simulink model "handone_simulink_2018b"  (R2018b)
settings: Solver=ode1  StartTime=0.0  StopTime=5  FixedStep=1e-3  RelTol=1e-3
model workspace: external: MAT-File D:\repos\hand_modeling_toolbox\examples\hand_one\hand_one_model.mat (data not in the file)
values from neighbouring files (symbols this model uses):
  d_coupling = 1e-5    (= 1e-05)    [hand_one_PTI.m]
  D_j = 1e-4 * [1,1,1,1]'    [hand_one_PTI.m]    (also in hand_one_model.m = 0* 1e-5 * [1,1,1,1]')
  finger_handone = init_from_rst(finger_urdf)    [hand_one_PTI.m]    (also in hand_one_model.m)
  k_coupling = 1e-1    (= 0.1)    [hand_one_PTI.m]
  mdh_matrix = mdh_struct_to_matrix(mdh_ori,1)    [create_handone_finger_from_urdf.m]    (also in hand_one_PTI.m; hand_one_model.m)
  q_init = [0.2,0.2]'    [create_hand_one_finger.m]    (also in hand_one_PTI.m = [0,0,0,0]'; hand_one_model.m = [0,0,0.1,0]')
  q_stiff_init = [0,0,0,0]'    [hand_one_PTI.m]    (also in hand_one_model.m)
  qD_init = [0,0,0,0]'    [hand_one_PTI.m]    (also in hand_one_model.m)
  S_j = 1e-4 * [1,1,1,1]'    [hand_one_PTI.m]    (also in hand_one_model.m = 0* 1e-4 * [1,1,1,1]')
undefined symbols (not defined in the file or in its folder): q_desired
libraries: unity_lib_UDP x1
settings Model: Creator=ge26jow  LastModifiedBy=ge26jow
settings DataIOCC: ReturnWorkspaceOutputs=on
settings DebuggingCC: SFMachineParentedDataDiag=error

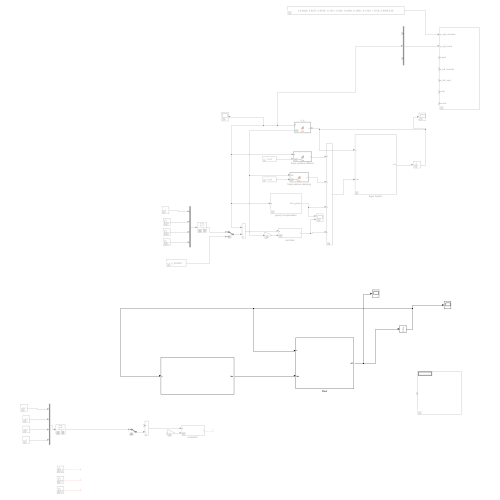
[thumbnail: Simulink's stored preview of the top-level diagram]
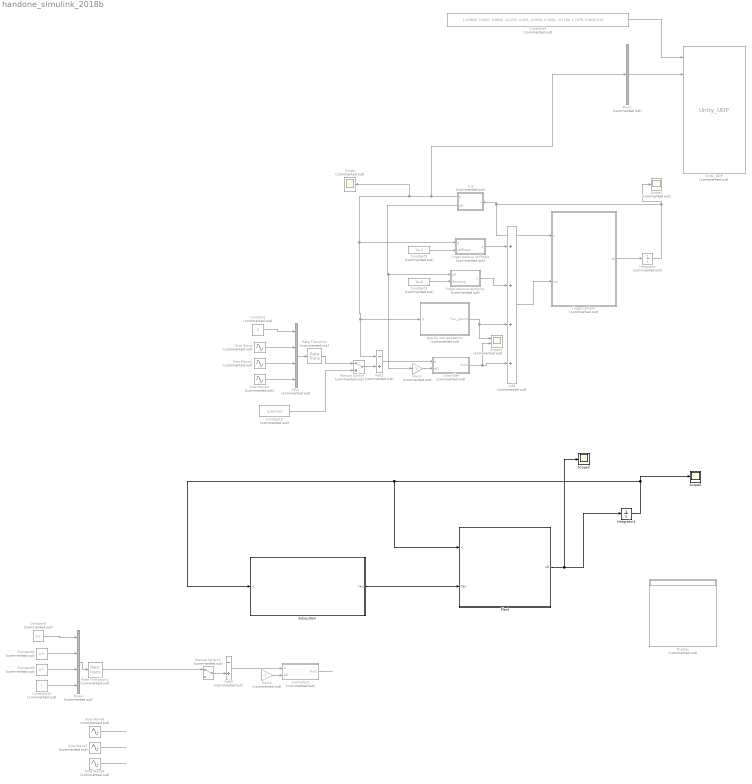
== system handone_simulink_2018b ==
  Add : Sum  Commented=on  Inputs=++++
  Add1 : Sum  Commented=on  Inputs=-+
  Add3 : Sum  Commented=on  Inputs=-+
  Constant : Constant  Commented=on  Value=0
  Constant1 : Constant  Commented=on  Value=1e-4
  Constant10 : Constant  Commented=on
  Constant2 : Constant  Commented=on  Value=1e-6
  Constant3 : Constant  Commented=on  Value=q_desired
  Constant4 : Constant  Commented=on  Value=[-0.3826, 0.0537, 0.0830, -0.1231, 0.435, -0.0500, 0.1060, -0.1700, 1.7279, 2.9845,0,0]'
  Constant5 : Constant  Commented=on  Value=0.2
  Constant8 : Constant  Commented=on  Value=0.5
  Constant9 : Constant  Commented=on  Value=0.7
  Display : Display  Commented=on
  Gain1 : Gain  Commented=on  Gain=-1
  Gain2 : Gain  Commented=on  Gain=-1
  Integrator : Integrator  Commented=on  InitialCondition=[q_init;qD_init]  WrappedStateUpperValue=[pi,pi,pi,pi,1e4,1e4,1e4,1e4]  WrappedStateLowerValue=-[pi,pi,pi,pi,1e4,1e4,1e4,1e4]
  Integrator1 : Integrator  InitialCondition=[q_init;qD_init]  WrappedStateUpperValue=[pi,pi,pi,pi,1e4,1e4,1e4,1e4]  WrappedStateLowerValue=-[pi,pi,pi,pi,1e4,1e4,1e4,1e4]
  Manual Switch : ManualSwitch  Commented=on
  Manual Switch1 : ManualSwitch  Commented=on
  Mux : Mux  Commented=on
  Mux1 : Mux  Commented=on  Inputs=[6,4,16]
  Mux2 : Mux  Commented=on
  Plant : Subsystem
  Rate Transition : RateTransition  Commented=on  OutPortSampleTime=1e-2
  Rate Transition1 : RateTransition  Commented=on  OutPortSampleTime=1e-2
  Scope : Scope  Commented=on
  Scope1 : Scope  Commented=on
  Scope2 : Scope  Commented=on  NumInputPorts=2
  Scope3 : Scope
  Scope5 : Scope
  Sine Wave{,1..2,6..8} (6 alike) : Sin  Commented=on  Amplitude=0.5  Bias=0.5
  Subsystem : Subsystem
  Unity_UDP : unity_lib_UDP/Unity_UDP  Commented=on  IP_port=8051  sampling_time=1e-2
  controller : Subsystem  Commented=on
  controller1 : Subsystem  Commented=on
  finger passive damping : MATLAB Function  Commented=on  TreatAsAtomicUnit=on
  finger passive stiffness : MATLAB Function  Commented=on  TreatAsAtomicUnit=on
  finger system : Subsystem  Commented=on
  gravity compensation : Subsystem  Commented=on
  x_q : MATLAB Function  Commented=on  TreatAsAtomicUnit=on
  wires:
  finger system/1(xd) -> Integrator/1
  x_q/1(q) -> Mux1/2, finger passive stiffness/1(q), Add1/1, gravity compensation/1(q), Scope/1
  Add/1 -> finger system/2(tau)
  finger passive stiffness/1(y) -> Add/1
  finger passive damping/1(y) -> Add/2
  x_q/2(qD) -> Gain1/1, finger passive damping/1(qD)
  Constant1/1 -> finger passive stiffness/2(stiffness)
  Constant2/1 -> finger passive damping/2(damping)
  gravity compensation/1(Tau_gravity) -> Add/3, Scope2/1
  Add1/1 -> controller/1(e)
  controller/1(Out1) -> Scope2/2, Add/4
  Gain1/1 -> controller/2(eD)
  Integrator/1 -> Scope1/1, x_q/1(u), finger system/1(x)
  Mux1/1 -> Unity_UDP/2
  Sine Wave/1 -> Mux/2
  Constant/1 -> Mux/1
  Sine Wave1/1 -> Mux/3
  Sine Wave2/1 -> Mux/4
  Manual Switch/1 -> Add1/2
  Constant3/1 -> Manual Switch/2
  Mux/1 -> Rate Transition/1
  Rate Transition/1 -> Manual Switch/1
  Constant4/1 -> Unity_UDP/1
  Add3/1 -> controller1/1(e)
  Constant5/1 -> Mux2/1
  Manual Switch1/1 -> Add3/2
  Mux2/1 -> Rate Transition1/1
  controller1/1(Out1) -> ?
  Gain2/1 -> controller1/2(eD)
  Rate Transition1/1 -> Manual Switch1/1
  Constant10/1 -> Mux2/4
  Constant8/1 -> Mux2/2
  Constant9/1 -> Mux2/3
  Sine Wave7/1 -> ?
  Sine Wave8/1 -> ?
  Sine Wave6/1 -> ?
  Integrator1/1 -> Scope5/1, Subsystem/1(x), Plant/1(x)
  Plant/1(xD) -> Scope3/1, Integrator1/1
  Subsystem/1(tau) -> Plant/2(tau)

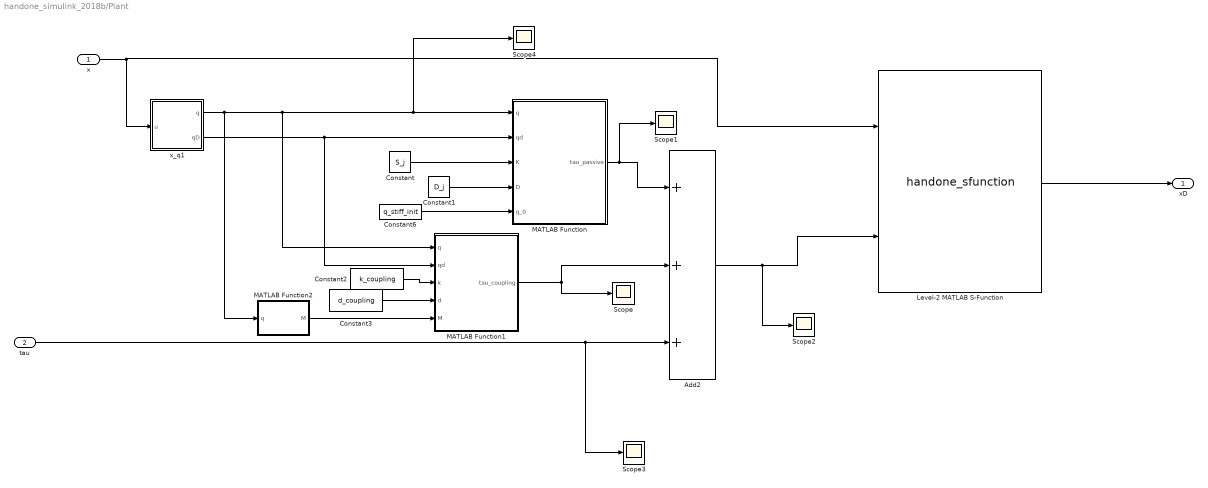
== system handone_simulink_2018b/Plant ==
  x : Inport
  tau : Inport  Port=2
  Add2 : Sum  Inputs=+++
  Constant : Constant  Value=S_j
  Constant1 : Constant  Value=D_j
  Constant2 : Constant  Value=k_coupling
  Constant3 : Constant  Value=d_coupling
  Constant6 : Constant  Value=q_stiff_init
  Level-2 MATLAB S-Function : M-S-Function  FunctionName=handone_sfunction
  MATLAB Function : MATLAB Function  TreatAsAtomicUnit=on
  MATLAB Function1 : MATLAB Function  TreatAsAtomicUnit=on
  MATLAB Function2 : MATLAB Function  TreatAsAtomicUnit=on
  Scope{,1..4} (5 alike) : Scope
  x_q1 : MATLAB Function  TreatAsAtomicUnit=on
  xD : Outport
  wires:
  Level-2 MATLAB S-Function/1 -> xD/1
  x/1 -> Level-2 MATLAB S-Function/1, x_q1/1(u)
  tau/1 -> Scope3/1, Add2/3
  Add2/1 -> Scope2/1, Level-2 MATLAB S-Function/2
  Constant6/1 -> MATLAB Function/5(q_0)
  x_q1/1(q) -> MATLAB Function2/1(q), MATLAB Function1/1(q), Scope4/1, MATLAB Function/1(q)
  x_q1/2(qD) -> MATLAB Function1/2(qd), MATLAB Function/2(qd)
  Constant/1 -> MATLAB Function/3(K)
  Constant1/1 -> MATLAB Function/4(D)
  MATLAB Function/1(tau_passive) -> Scope1/1, Add2/1
  MATLAB Function1/1(tau_coupling) -> Add2/2, Scope/1
  Constant2/1 -> MATLAB Function1/3(k)
  MATLAB Function2/1(M) -> MATLAB Function1/5(M)
  Constant3/1 -> MATLAB Function1/4(d)

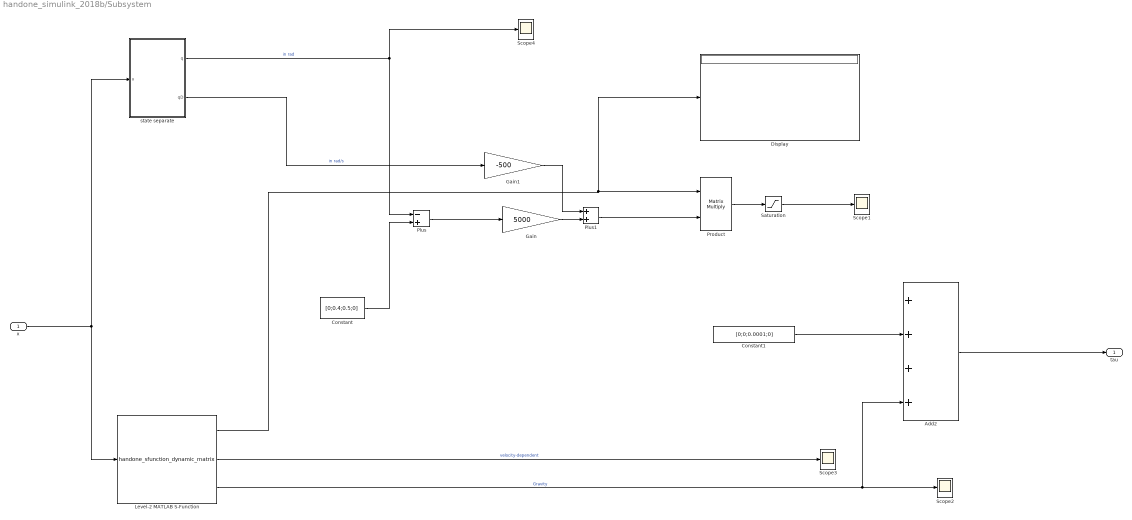
== system handone_simulink_2018b/Subsystem ==
  x : Inport
  Add2 : Sum  Inputs=++++
  Constant : Constant  Value=[0;0.4;0.5;0]  VectorParams1D=off
  Constant1 : Constant  Value=[0;0;0.0001;0]
  Display : Display
  Gain : Gain  Gain=5000
  Gain1 : Gain  Gain=-500
  Level-2 MATLAB S-Function : M-S-Function  FunctionName=handone_sfunction_dynamic_matrix
  Plus : Sum  Inputs=-+
  Plus1 : Sum
  Product : Product  Multiplication=Matrix(*)
  Saturation : Saturate  UpperLimit=5e-3  LowerLimit=-5e-3
  Scope{1..4} (4 alike) : Scope
  state separate : MATLAB Function  TreatAsAtomicUnit=on
  tau : Outport
  wires:
  state separate/1(q) -> Plus/1, Scope4/1  "in rad"
  x/1 -> state separate/1(u), Level-2 MATLAB S-Function/1
  Level-2 MATLAB S-Function/1 -> Display/1, Product/1
  Level-2 MATLAB S-Function/2 -> Scope3/1  "velocity-dependent"
  Level-2 MATLAB S-Function/3 -> Add2/4, Scope2/1  "Gravity"
  Product/1 -> Saturation/1
  Constant/1 -> Plus/2
  Plus/1 -> Gain/1
  Gain/1 -> Plus1/2
  Gain1/1 -> Plus1/1
  state separate/2(qD) -> Gain1/1  "in rad/s"
  Plus1/1 -> Product/2
  Saturation/1 -> Scope1/1
  Add2/1 -> tau/1
  Constant1/1 -> Add2/2

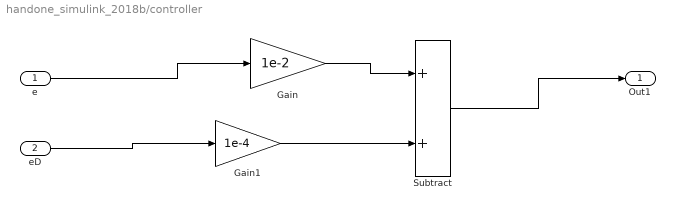
== system handone_simulink_2018b/controller ==
  e : Inport
  eD : Inport  Port=2
  Gain : Gain  Gain=1e-2
  Gain1 : Gain  Gain=1e-4
  Subtract : Sum
  Out1 : Outport
  wires:
  e/1 -> Gain/1
  Gain/1 -> Subtract/1
  eD/1 -> Gain1/1
  Gain1/1 -> Subtract/2
  Subtract/1 -> Out1/1

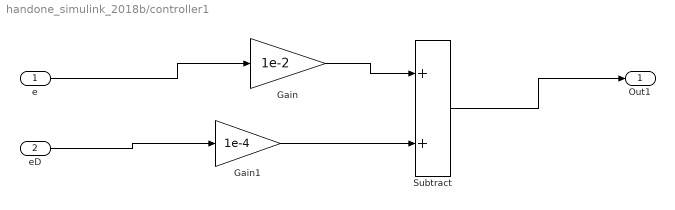
== system handone_simulink_2018b/controller1 ==
  e : Inport
  eD : Inport  Port=2
  Gain : Gain  Gain=1e-2
  Gain1 : Gain  Gain=1e-4
  Subtract : Sum
  Out1 : Outport
  wires:
  e/1 -> Gain/1
  Gain/1 -> Subtract/1
  eD/1 -> Gain1/1
  Gain1/1 -> Subtract/2
  Subtract/1 -> Out1/1

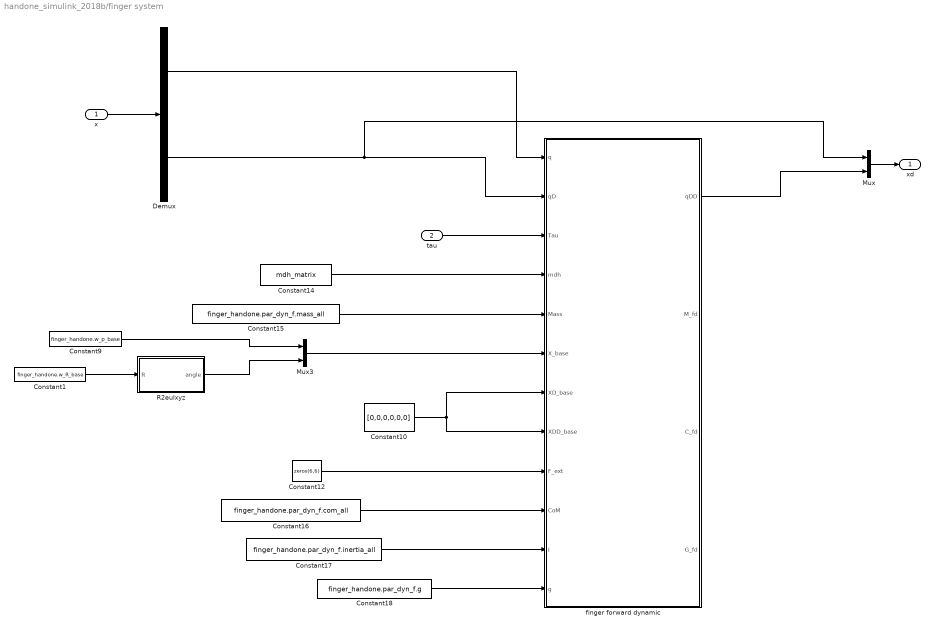
== system handone_simulink_2018b/finger system ==
  x : Inport  PortDimensions=8
  tau : Inport  Port=2
  Constant1 : Constant  Value=finger_handone.w_R_base
  Constant10 : Constant  Value=[0,0,0,0,0,0]
  Constant12 : Constant  Value=zeros(6,6)
  Constant14 : Constant  Value=mdh_matrix
  Constant15 : Constant  Value=finger_handone.par_dyn_f.mass_all
  Constant16 : Constant  Value=finger_handone.par_dyn_f.com_all
  Constant17 : Constant  Value=finger_handone.par_dyn_f.inertia_all
  Constant18 : Constant  Value=finger_handone.par_dyn_f.g
  Constant9 : Constant  Value=finger_handone.w_p_base
  Demux : Demux  Outputs=[4,4]
  Mux : Mux  Inputs=2
  Mux3 : Mux  Inputs=[3,3]
  R2eulxyz : MATLAB Function  TreatAsAtomicUnit=on
  finger forward dynamic : MATLAB Function  TreatAsAtomicUnit=on
  xd : Outport
  wires:
  Constant18/1 -> finger forward dynamic/12(g)
  tau/1 -> finger forward dynamic/3(Tau)
  Constant17/1 -> finger forward dynamic/11(I)
  finger forward dynamic/1(qDD) -> Mux/2
  Constant10/1 -> finger forward dynamic/7(XD_base), finger forward dynamic/8(XDD_base)
  Demux/2 -> Mux/1, finger forward dynamic/2(qD)
  Mux3/1 -> finger forward dynamic/6(X_base)
  Constant14/1 -> finger forward dynamic/4(mdh)
  Demux/1 -> finger forward dynamic/1(q)
  Constant12/1 -> finger forward dynamic/9(F_ext)
  Constant15/1 -> finger forward dynamic/5(Mass)
  Constant16/1 -> finger forward dynamic/10(CoM)
  Mux/1 -> xd/1
  x/1 -> Demux/1
  Constant1/1 -> R2eulxyz/1(R)
  R2eulxyz/1(angle) -> Mux3/2
  Constant9/1 -> Mux3/1

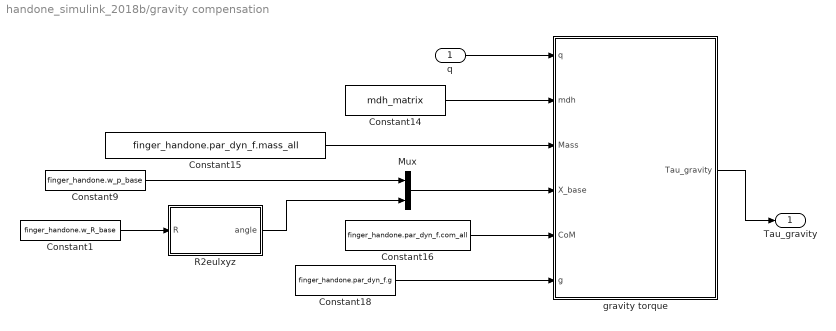
== system handone_simulink_2018b/gravity compensation ==
  q : Inport
  Constant1 : Constant  Value=finger_handone.w_R_base
  Constant14 : Constant  Value=mdh_matrix
  Constant15 : Constant  Value=finger_handone.par_dyn_f.mass_all
  Constant16 : Constant  Value=finger_handone.par_dyn_f.com_all
  Constant18 : Constant  Value=finger_handone.par_dyn_f.g
  Constant9 : Constant  Value=finger_handone.w_p_base
  Mux : Mux  Inputs=[3,3]
  R2eulxyz : MATLAB Function  TreatAsAtomicUnit=on
  "gravity torque " : MATLAB Function  TreatAsAtomicUnit=on
  Tau_gravity : Outport
  wires:
  Constant14/1 -> "gravity torque "/2(mdh)
  Constant16/1 -> "gravity torque "/5(CoM)
  Mux/1 -> "gravity torque "/4(X_base)
  Constant18/1 -> "gravity torque "/6(g)
  Constant15/1 -> "gravity torque "/3(Mass)
  "gravity torque "/1(Tau_gravity) -> Tau_gravity/1
  q/1 -> "gravity torque "/1(q)
  Constant1/1 -> R2eulxyz/1(R)
  Constant9/1 -> Mux/1
  R2eulxyz/1(angle) -> Mux/2

== matlab function handone_simulink_2018b/x_q ==
  data: u input; q output; qD output
function [q,qD] = fcn(u)

q = u(1:4);
qD = u(5:8);

== matlab function handone_simulink_2018b/finger system/finger forward dynamic ==
  data: q input; qDD output; qD input; Tau input; mdh input; Mass input; X_base input; XD_base input; XDD_base input; F_ext input; CoM input; I input; g input; M_fd output; C_fd output; G_fd output
% recursive Newton-Euler method to compute inverse dynamic with mdh
% parameters
% Input:
%     q,qD:             [n_qx1] joint states
%     Tau               [n_q] joint torque
%     mdh:              [n_q+1x4] in sequence of [alpha,a,theta,d] To be
%                       noted that the theta should exclude from mdh parameters 
%     Mass:             [n_q+1] mass vector. the first mass is the base 
%     X_base:           [6x1] eulerxyz
%     XD_base:          [6x1] translational and angular velocity
%     F_ext:            [6x1] force/moment that exerted by the environment to the endeffector frame. 
%     CoM:              [3xn_q+1] in local frame; last column is endeffector
%     I:                [6xn_q+1] in local frame with respect to center of mass. in sequence of [xx yy zz yz xz xy]
%     g:                [3x1] gravity term
% 
% Output:
%     qDD:              [n_qx1] joint acceleration 
%     M_fd:             [n_qxn_q] Mass matrix 
%     C_fd:             [n_q] velocity-dependent torque 
%     G_fd:             [n_q] gravity torque  

function [qDD,M_fd,C_fd,G_fd] = fordyn_ne_mdh(q,qD,Tau,mdh, Mass, X_base, XD_base,XDD_base, F_ext, CoM, I, g)
coder.extrinsic('invdyn_ne_mdh_mex');

n_q = length(q);
% assert(n_q == length(qD)&&n_q == length(Tau),'fordyn_ne_mdh: dimension error!');

mex = 1;


M_fd = zeros(n_q,n_q);
G_fd = zeros(n_q,1);
C_fd = zeros(n_q,1);

% gravity term
if mex
    G_fd = invdyn_ne_mdh_mex(q,zeros(n_q,1),zeros(n_q,1),mdh, Mass,...
        X_base, XD_base, XDD_base, zeros(6,1), CoM, I, g);
else
    G_fd = invdyn_ne_mdh(q,zeros(n_q,1),zeros(n_q,1),mdh, Mass,...
        X_base, XD_base, XDD_base, zeros(6,1), CoM, I, g);
end
% C term
if mex
    C_fd = invdyn_ne_mdh_mex(q,qD,zeros(n_q,1),mdh, Mass,...
        X_base, XD_base, XDD_base, zeros(6,1), CoM, I, g);
else
    C_fd = invdyn_ne_mdh(q,qD,zeros(n_q,1),mdh, Mass,...
             X_base, XD_base, XDD_base, zeros(6,1), CoM, I, g);
end
C_fd = C_fd - G_fd;

% M term
M_fd = zeros(n_q,n_q);

for i = 1:n_q
    qDD_M = zeros(n_q,1);
    qDD_M(i) = 1;
    if mex
        M_fd(:,i) = invdyn_ne_mdh_mex(q,zeros(n_q,1),qDD_M,mdh, Mass,...
            X_base, XD_base, XDD_base, zeros(6,1), CoM, I, g);
    else
        M_fd(:,i) = invdyn_ne_mdh(q,zeros(n_q,1),qDD_M,mdh, Mass,...
            X_base, XD_base, XDD_base, zeros(6,1), CoM, I, g);
    end
    M_fd(:,i) = M_fd(:,i) - G_fd;
end

% use Jacobian_geom_mdh.m to calculate geometric Jacobian
w_R_b = euler2R_XYZ(X_base(4:6));
b_J = Jacobian_geom_mdh(mdh,q);
J_ne = blkdiag(w_R_b,w_R_b)*b_J;
tau_ext = zeros(n_q,1);
for i = 1:n_q+1
    mdh_i = mdh(1:i,:);
    q_i = q(1:min(i,n_q));
    b_J_i = zeros(6,n_q);
    b_J_i(:,1:min(i,n_q)) =  Jacobian_geom_mdh(mdh_i,q_i);
    J_ne_i= blkdiag(w_R_b,w_R_b)*b_J_i;
    tau_i = J_ne_i'*F_ext(:,i+1);
    tau_ext = tau_ext + tau_i;
end


qDD = (M_fd)\(Tau + tau_ext - G_fd - C_fd);


end

== matlab function handone_simulink_2018b/finger passive stiffness ==
  data: q input; y output; stiffness input
function y = fcn(q,stiffness)

y = -stiffness.*q;

== matlab function handone_simulink_2018b/finger passive damping ==
  data: qD input; y output; damping input
function y = fcn(qD,damping)

y = -damping.*qD;

== matlab function handone_simulink_2018b/gravity compensation/gravity torque  ==
  data: q input; Tau_gravity output; mdh input; Mass input; X_base input; CoM input; g input
function Tau_gravity = fcn(q,mdh, Mass, X_base, CoM, g)

Tau_gravity = invdyn_ne_mdh_all_fext_gravity(q,mdh, Mass, X_base, CoM, g);

== matlab function handone_simulink_2018b/gravity compensation/R2eulxyz ==
  data: R input; angle output
function angle = fcn(R)

angle = R2euler_XYZ(R);

== matlab function handone_simulink_2018b/finger system/R2eulxyz ==
  data: R input; angle output
function angle = fcn(R)

angle = R2euler_XYZ(R);

== matlab function handone_simulink_2018b/Plant/MATLAB Function ==
  data: q input; tau_passive output; qd input; K input; D input; q_0 input
function tau_passive = passive_torque(q,qd,K,D,q_0)

tau_passive = K.*(q_0 - q) - D.*(qd);

== matlab function handone_simulink_2018b/Plant/MATLAB Function1 ==
  data: q input; qd input; tau_coupling output; k input; d input; M input
function tau_coupling = coupling_torque(q,qd,k,d,M)
tau_coupling = zeros(size(q));
delta_l = M(3)*q(3) - M(4)*q(4);
delta_ld = M(3)*qd(3) - M(4)*qd(4);
if delta_l > 0
    tau_coupling = [0;0;-k;k]*delta_l - [0;0;d;-d]*delta_ld;
else
    tau_coupling = zeros(size(q));
end

== matlab function handone_simulink_2018b/Plant/MATLAB Function2 ==
  data: q input; M output
function M = moment_arm(q)

M = 0.01*ones(size(q));

== matlab function handone_simulink_2018b/Subsystem/state separate ==
  data: u input; q output; qD output
function [q,qD] = fcn(u)

q = u(1:4);
qD = u(5:8);

== matlab function handone_simulink_2018b/Plant/x_q1 ==
  data: u input; q output; qD output
function [q,qD] = fcn(u)

q = u(1:4);
qD = u(5:8);
